simulink model "WP1CicloChiuso"  (R2023b)
settings: Solver=VariableStepAuto  StartTime=0.0  StopTime=10  RelTol=1e-10
values from neighbouring files (symbols this model uses):
  K = [18235, 53.9]    [CicloChiuso.m]
  r = pi    (= 3.14159265359)    [CicloChiuso.m]
undefined symbols (not defined in the file or in its folder): Kr, r_nl, u_e, x_e
settings Model: Creator=franc  LastModifiedBy=beniaminosquitieri

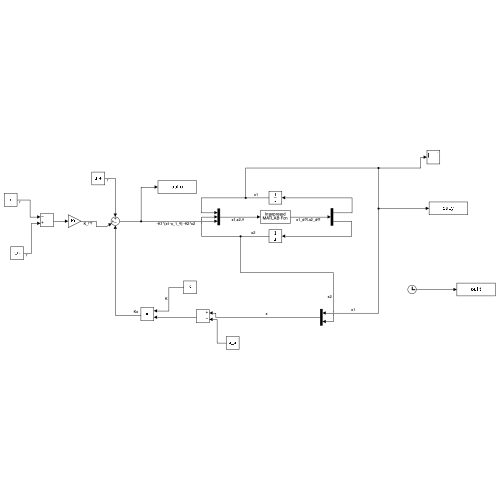
[thumbnail: Simulink's stored preview of the top-level diagram]
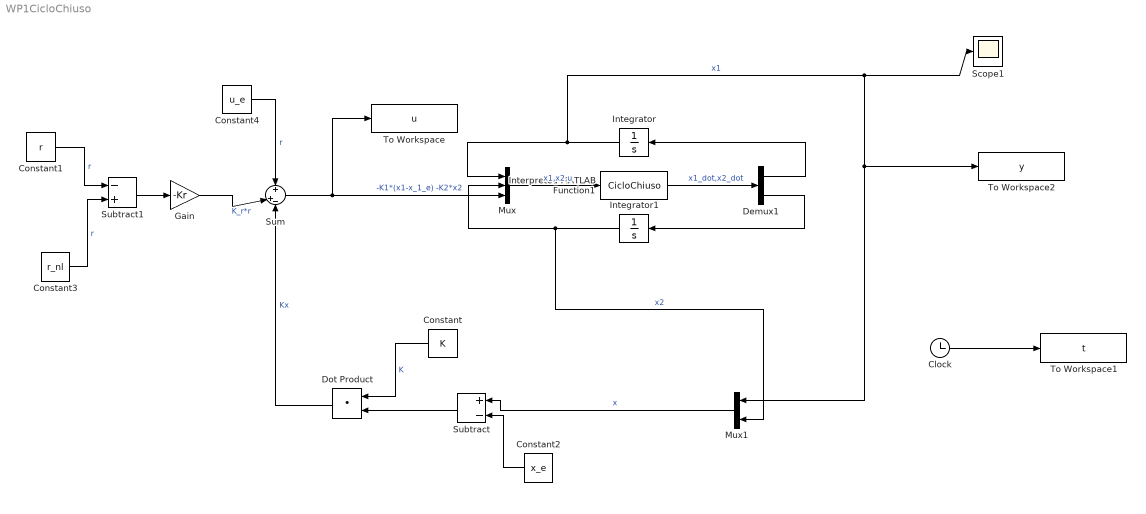
== system WP1CicloChiuso ==
  Clock : Clock
  Constant : Constant  Value=K
  Constant1 : Constant  Value=r
  Constant2 : Constant  Value=x_e
  Constant3 : Constant  Value=r_nl
  Constant4 : Constant  Value=u_e
  Demux1 : Demux  Outputs=2
  Dot Product : DotProduct  OutDataTypeStr=Inherit: Inherit via internal rule
  Gain : Gain  Gain=-Kr
  Integrator : Integrator
  Integrator1 : Integrator
  Interpreted MATLAB Function1 : MATLABFcn  MATLABFcn=CicloChiuso  OutputDimensions=2
  Mux : Mux  Inputs=3
  Mux1 : Mux  Inputs=2
  Scope1 : Scope
  Subtract : Sum  Inputs=+-
  Subtract1 : Sum  Inputs=-+
  Sum : Sum  Inputs=+|+-
  To Workspace : ToWorkspace  VariableName=u  SampleTime=-1
  To Workspace1 : ToWorkspace  VariableName=t  SampleTime=-1
  To Workspace2 : ToWorkspace  VariableName=y  SampleTime=-1
  wires:
  Interpreted MATLAB Function1/1 -> Demux1/1  "x1_dot,x2_dot"
  Constant/1 -> Dot Product/1  "K"
  Demux1/2 -> Integrator1/1
  Demux1/1 -> Integrator/1
  Mux/1 -> Interpreted MATLAB Function1/1  "x1,x2,u"
  Integrator/1 -> Scope1/1, To Workspace2/1, Mux1/1, Mux/1  "x1"
  Integrator1/1 -> Mux1/2, Mux/2  "x2"
  Clock/1 -> To Workspace1/1
  Mux1/1 -> Subtract/1  "x"
  Constant2/1 -> Subtract/2
  Subtract/1 -> Dot Product/2
  Sum/1 -> To Workspace/1, Mux/3  "-K1*(x1-x_1_e) -K2*x2"
  Constant3/1 -> Subtract1/2  "r"
  Constant1/1 -> Subtract1/1  "r"
  Subtract1/1 -> Gain/1
  Constant4/1 -> Sum/1  "r"
  Dot Product/1 -> Sum/3  "Kx"
  Gain/1 -> Sum/2  "K_r*r"
